simulink model "controller_AWBT"  (R2015a)
settings: Solver=ode5  StartTime=0.0  StopTime=6  FixedStep=1e-4  RelTol=1e-3
values from neighbouring files (symbols this model uses):
  H = [5.12681187314e-07 0.112742656092 2.44237784514e-07 -0.105533295669]    [additional.mat]
  J = [2.83860804855e-05  -1.6026480482e-05; 10.5960240586  -0.732650067931; 1.35229331217e-05  -7.63490485575e-06; 13.4258430852  -0.928315474954]    [additional.mat]
  L = [-25.7541759314 0.409811538959 3.06306499805 0.254874011741]    [additional.mat]
  Lambda = X/M    [second_phase.m]
  Lambda_LQG = X/M    [second_phase.m]
  N = [0.000228245301669 -37.0804932344 0.000108734488772 -46.9833485255 221.436555387 -2.86027336512 -16.0597823804 -2.25808078226 -0.000990896933621 -217.906088567 -0.00047205647045 -276.101033302 ... (16 elements, 4x4)]    [additional.mat]
undefined symbols (not defined in the file or in its folder): Ap, Bp, Cp, Hp, Lest
libraries: cstblocks x4, simulink x1
settings Model: Creator=p4wp4w  LastModifiedBy=p4wp4w
settings SolverCC: AlgebraicLoopSolver=LineSearch

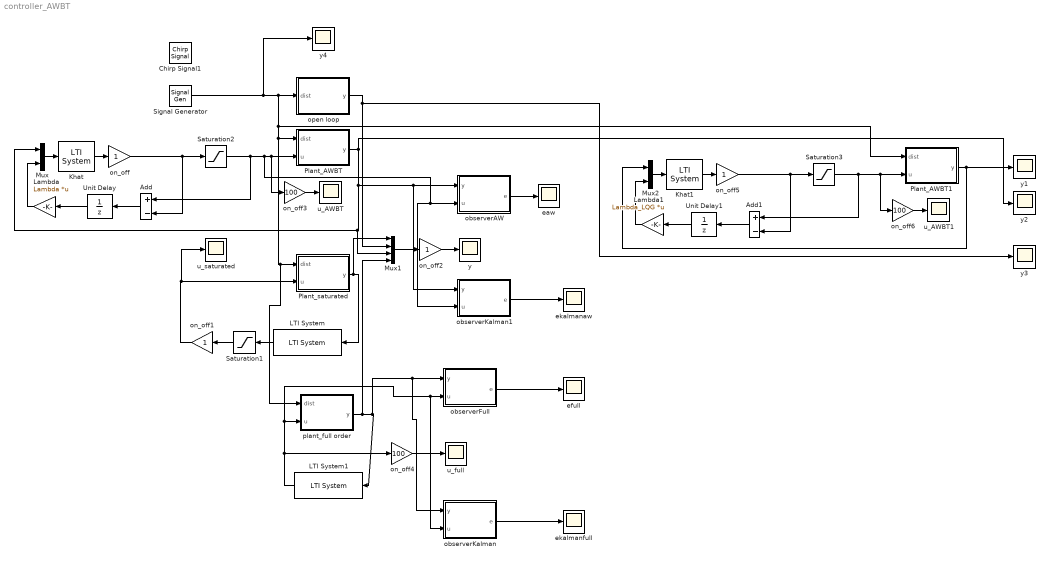
== system controller_AWBT ==
  Add : Sum  Inputs=+-
  Add1 : Sum  Inputs=+-
  Chirp Signal1 : simulink/Sources/Chirp Signal  f1=0.1  T=9  f2=90
  Khat : cstblocks/LTI System  sys=Khat  IC=[]
  Khat1 : cstblocks/LTI System  sys=Khat_LQG  IC=[]
  LTI System : cstblocks/LTI System  sys=controller_implemented  IC=[]
  LTI System1 : cstblocks/LTI System  sys=controller_implemented  IC=[]
  Lambda : Gain  Gain=Lambda  Multiplication=Matrix(K*u)
  Lambda1 : Gain  Gain=Lambda_LQG  Multiplication=Matrix(K*u)
  Mux : Mux  Inputs=2
  Mux1 : Mux
  Mux2 : Mux  Inputs=2
  Plant_AWBT : Subsystem
  Plant_AWBT1 : Subsystem
  Plant_saturated : Subsystem
  Saturation1 : Saturate  UpperLimit=1.5  LowerLimit=-1.5
  Saturation2 : Saturate  UpperLimit=1.5  LowerLimit=-1.5
  Saturation3 : Saturate  UpperLimit=1.5  LowerLimit=-1.5
  Signal Generator : SignalGenerator  WaveForm=square  Frequency=2  Units=rad/sec
  Unit Delay : UnitDelay  SampleTime=-1
  Unit Delay1 : UnitDelay  SampleTime=-1
  eaw : Scope
      settings: ShowLegends=on  YMin=-4  YMax=4  SaveName=eaw
  efull : Scope
      settings: ShowLegends=on  YMin=-4  YMax=4  SaveName=efull
  ekalmanaw : Scope
      settings: ShowLegends=on  YMin=-4  YMax=4  SaveName=efull2
  ekalmanfull : Scope
      settings: ShowLegends=on  YMin=-4  YMax=4  SaveName=ekalman
  observerAW : Subsystem
  observerFull : Subsystem
  observerKalman : Subsystem
  observerKalman1 : Subsystem
  on_off{,1..2,5} (4 alike) : Gain
  on_off3 : Gain  Gain=100
  on_off4 : Gain  Gain=100
  on_off6 : Gain  Gain=100
  open loop : Subsystem
  plant_full order : Subsystem
  u_AWBT : Scope
      settings: YMin=-0.75  YMax=0.75  SaveName=uaw
  u_AWBT1 : Scope
      settings: YMin=-0.75  YMax=0.75  SaveName=uaw_lqg
  u_full : Scope
      settings: SaveName=ufull
  u_saturated : Scope
      settings: SaveName=ScopeData2
  y{,1..4} (5 alike) : Scope
      y settings: ShowLegends=on  YMin=-4  YMax=4  SaveName=output
      y1 settings: ShowLegends=on  YMin=-4  YMax=4  SaveName=output_lqg
      y2 settings: ShowLegends=on  YMin=-4  YMax=4  SaveName=output_aw
      y3 settings: ShowLegends=on  YMin=-4  YMax=4  SaveName=output_open
      y4 settings: ShowLegends=on  YMin=-4  YMax=4  SaveName=dist
  wires:
  Mux/1 -> Khat/1
  Plant_AWBT/1(y) -> observerKalman1/1(y), observerAW/1(y), Mux1/3, Mux/1, y2/1
  Khat/1 -> on_off/1
  LTI System/1 -> Saturation1/1
  Plant_saturated/1(y) -> LTI System/1, Mux1/1
  Saturation1/1 -> on_off1/1
  Mux1/1 -> on_off2/1
  on_off1/1 -> u_saturated/1, Plant_saturated/2(u)
  Lambda/1 -> Mux/2
  on_off/1 -> Add/2, Saturation2/1
  Saturation2/1 -> Add/1, observerAW/2(u), observerKalman1/2(u), on_off3/1, Plant_AWBT/2(u)
  Add/1 -> Unit Delay/1
  Unit Delay/1 -> Lambda/1
  LTI System1/1 -> observerKalman/2(u), observerFull/2(u), plant_full order/2(u), on_off4/1
  plant_full order/1(y) -> Mux1/4, observerKalman/1(y), observerFull/1(y), LTI System1/1
  on_off2/1 -> y/1
  on_off3/1 -> u_AWBT/1
  on_off4/1 -> u_full/1
  observerAW/1(e) -> eaw/1
  observerFull/1(e) -> efull/1
  observerKalman/1(e) -> ekalmanfull/1
  observerKalman1/1(e) -> ekalmanaw/1
  Mux2/1 -> Khat1/1
  Plant_AWBT1/1(y) -> y1/1, Mux2/1
  Khat1/1 -> on_off5/1
  Lambda1/1 -> Mux2/2
  on_off5/1 -> Saturation3/1, Add1/2
  Saturation3/1 -> Plant_AWBT1/2(u), on_off6/1, Add1/1
  Signal Generator/1 -> y4/1, Plant_AWBT1/1(dist), plant_full order/1(dist), Plant_saturated/1(dist), Plant_AWBT/1(dist), open loop/1(dist)
  on_off6/1 -> u_AWBT1/1
  Add1/1 -> Unit Delay1/1
  open loop/1(y) -> y3/1, Mux1/2
  Unit Delay1/1 -> Lambda1/1

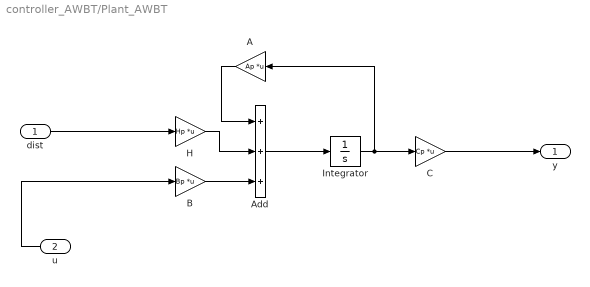
== system controller_AWBT/Plant_AWBT ==
  dist : Inport
  u : Inport  Port=2
  A : Gain  Gain=Ap  Multiplication=Matrix(K*u)
  Add : Sum  Inputs=+++
  B : Gain  Gain=Bp  Multiplication=Matrix(K*u)
  C : Gain  Gain=Cp  Multiplication=Matrix(K*u)
  H : Gain  Gain=Hp  Multiplication=Matrix(K*u)
  Integrator : Integrator
  y : Outport
  wires:
  Add/1 -> Integrator/1
  H/1 -> Add/2
  A/1 -> Add/1
  dist/1 -> H/1
  B/1 -> Add/3
  Integrator/1 -> C/1, A/1
  u/1 -> B/1
  C/1 -> y/1

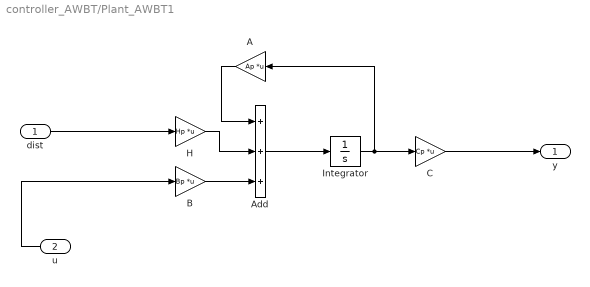
== system controller_AWBT/Plant_AWBT1 ==
  dist : Inport
  u : Inport  Port=2
  A : Gain  Gain=Ap  Multiplication=Matrix(K*u)
  Add : Sum  Inputs=+++
  B : Gain  Gain=Bp  Multiplication=Matrix(K*u)
  C : Gain  Gain=Cp  Multiplication=Matrix(K*u)
  H : Gain  Gain=Hp  Multiplication=Matrix(K*u)
  Integrator : Integrator
  y : Outport
  wires:
  C/1 -> y/1
  u/1 -> B/1
  Integrator/1 -> A/1, C/1
  B/1 -> Add/3
  dist/1 -> H/1
  A/1 -> Add/1
  H/1 -> Add/2
  Add/1 -> Integrator/1

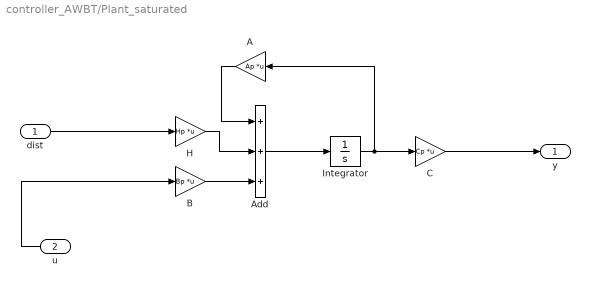
== system controller_AWBT/Plant_saturated ==
  dist : Inport
  u : Inport  Port=2
  A : Gain  Gain=Ap  Multiplication=Matrix(K*u)
  Add : Sum  Inputs=+++
  B : Gain  Gain=Bp  Multiplication=Matrix(K*u)
  C : Gain  Gain=Cp  Multiplication=Matrix(K*u)
  H : Gain  Gain=Hp  Multiplication=Matrix(K*u)
  Integrator : Integrator
  y : Outport
  wires:
  u/1 -> B/1
  Integrator/1 -> A/1, C/1
  B/1 -> Add/3
  dist/1 -> H/1
  A/1 -> Add/1
  H/1 -> Add/2
  Add/1 -> Integrator/1
  C/1 -> y/1

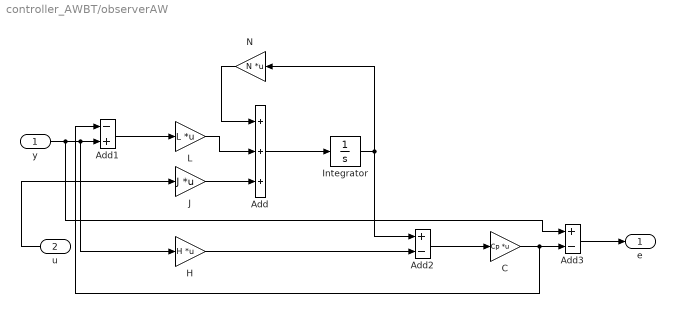
== system controller_AWBT/observerAW ==
  y : Inport
  u : Inport  Port=2
  Add : Sum  Inputs=+++
  Add1 : Sum  Inputs=-+
  Add2 : Sum  Inputs=+-
  Add3 : Sum  Inputs=+-
  C : Gain  Gain=Cp  Multiplication=Matrix(K*u)
  H : Gain  Gain=H  Multiplication=Matrix(K*u)
  Integrator : Integrator
  J : Gain  Gain=J  Multiplication=Matrix(K*u)
  L : Gain  Gain=L  Multiplication=Matrix(K*u)
  N : Gain  Gain=N  Multiplication=Matrix(K*u)
  e : Outport
  wires:
  Add/1 -> Integrator/1
  L/1 -> Add/2
  N/1 -> Add/1
  J/1 -> Add/3
  Integrator/1 -> Add2/1, N/1
  u/1 -> J/1
  y/1 -> Add3/1, H/1, Add1/2
  Add1/1 -> L/1
  H/1 -> Add2/2
  Add2/1 -> C/1
  C/1 -> Add1/1, Add3/2
  Add3/1 -> e/1

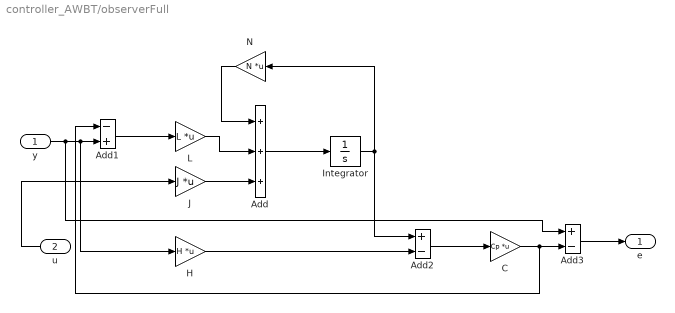
== system controller_AWBT/observerFull ==
  y : Inport
  u : Inport  Port=2
  Add : Sum  Inputs=+++
  Add1 : Sum  Inputs=-+
  Add2 : Sum  Inputs=+-
  Add3 : Sum  Inputs=+-
  C : Gain  Gain=Cp  Multiplication=Matrix(K*u)
  H : Gain  Gain=H  Multiplication=Matrix(K*u)
  Integrator : Integrator
  J : Gain  Gain=J  Multiplication=Matrix(K*u)
  L : Gain  Gain=L  Multiplication=Matrix(K*u)
  N : Gain  Gain=N  Multiplication=Matrix(K*u)
  e : Outport
  wires:
  Add3/1 -> e/1
  C/1 -> Add3/2, Add1/1
  Add2/1 -> C/1
  H/1 -> Add2/2
  Add1/1 -> L/1
  y/1 -> Add1/2, H/1, Add3/1
  u/1 -> J/1
  Integrator/1 -> N/1, Add2/1
  J/1 -> Add/3
  N/1 -> Add/1
  L/1 -> Add/2
  Add/1 -> Integrator/1

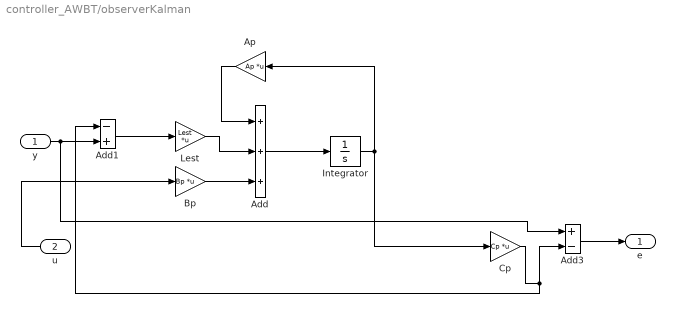
== system controller_AWBT/observerKalman ==
  y : Inport
  u : Inport  Port=2
  Add : Sum  Inputs=+++
  Add1 : Sum  Inputs=-+
  Add3 : Sum  Inputs=+-
  Ap : Gain  Gain=Ap  Multiplication=Matrix(K*u)
  Bp : Gain  Gain=Bp  Multiplication=Matrix(K*u)
  Cp : Gain  Gain=Cp  Multiplication=Matrix(K*u)
  Integrator : Integrator
  Lest : Gain  Gain=Lest  Multiplication=Matrix(K*u)
  e : Outport
  wires:
  Add/1 -> Integrator/1
  Lest/1 -> Add/2
  Ap/1 -> Add/1
  Bp/1 -> Add/3
  Integrator/1 -> Ap/1, Cp/1
  u/1 -> Bp/1
  y/1 -> Add3/1, Add1/2
  Add1/1 -> Lest/1
  Cp/1 -> Add3/2, Add1/1
  Add3/1 -> e/1

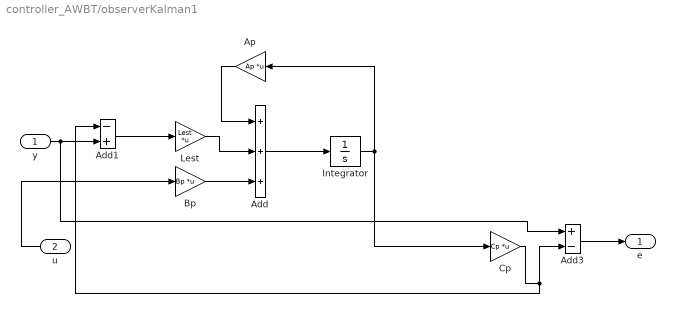
== system controller_AWBT/observerKalman1 ==
  y : Inport
  u : Inport  Port=2
  Add : Sum  Inputs=+++
  Add1 : Sum  Inputs=-+
  Add3 : Sum  Inputs=+-
  Ap : Gain  Gain=Ap  Multiplication=Matrix(K*u)
  Bp : Gain  Gain=Bp  Multiplication=Matrix(K*u)
  Cp : Gain  Gain=Cp  Multiplication=Matrix(K*u)
  Integrator : Integrator
  Lest : Gain  Gain=Lest  Multiplication=Matrix(K*u)
  e : Outport
  wires:
  Add3/1 -> e/1
  Cp/1 -> Add1/1, Add3/2
  Add1/1 -> Lest/1
  y/1 -> Add1/2, Add3/1
  u/1 -> Bp/1
  Integrator/1 -> Cp/1, Ap/1
  Bp/1 -> Add/3
  Ap/1 -> Add/1
  Lest/1 -> Add/2
  Add/1 -> Integrator/1

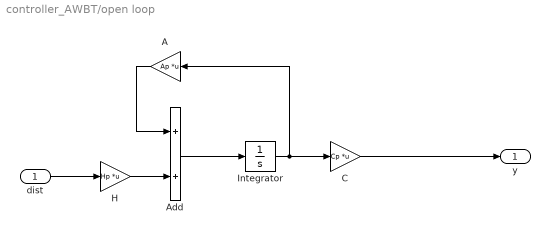
== system controller_AWBT/open loop ==
  dist : Inport
  A : Gain  Gain=Ap  Multiplication=Matrix(K*u)
  Add : Sum
  C : Gain  Gain=Cp  Multiplication=Matrix(K*u)
  H : Gain  Gain=Hp  Multiplication=Matrix(K*u)
  Integrator : Integrator
  y : Outport
  wires:
  Integrator/1 -> A/1, C/1
  dist/1 -> H/1
  A/1 -> Add/1
  H/1 -> Add/2
  Add/1 -> Integrator/1
  C/1 -> y/1

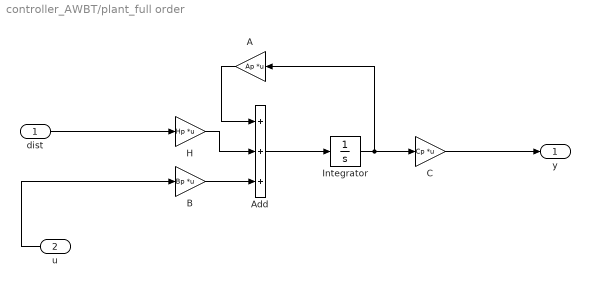
== system controller_AWBT/plant_full order ==
  dist : Inport
  u : Inport  Port=2
  A : Gain  Gain=Ap  Multiplication=Matrix(K*u)
  Add : Sum  Inputs=+++
  B : Gain  Gain=Bp  Multiplication=Matrix(K*u)
  C : Gain  Gain=Cp  Multiplication=Matrix(K*u)
  H : Gain  Gain=Hp  Multiplication=Matrix(K*u)
  Integrator : Integrator
  y : Outport
  wires:
  C/1 -> y/1
  Add/1 -> Integrator/1
  H/1 -> Add/2
  A/1 -> Add/1
  dist/1 -> H/1
  B/1 -> Add/3
  Integrator/1 -> C/1, A/1
  u/1 -> B/1
